simulink model "InverseKinematicsRefMod"  (R2016b)
settings: Solver=VariableStepAuto  StartTime=0.0  StopTime=10.0  RelTol=1e-3
settings Model: DataDictionary=DataDictionary.sldd  Creator=lucadelaat  LastModifiedBy=Taeke

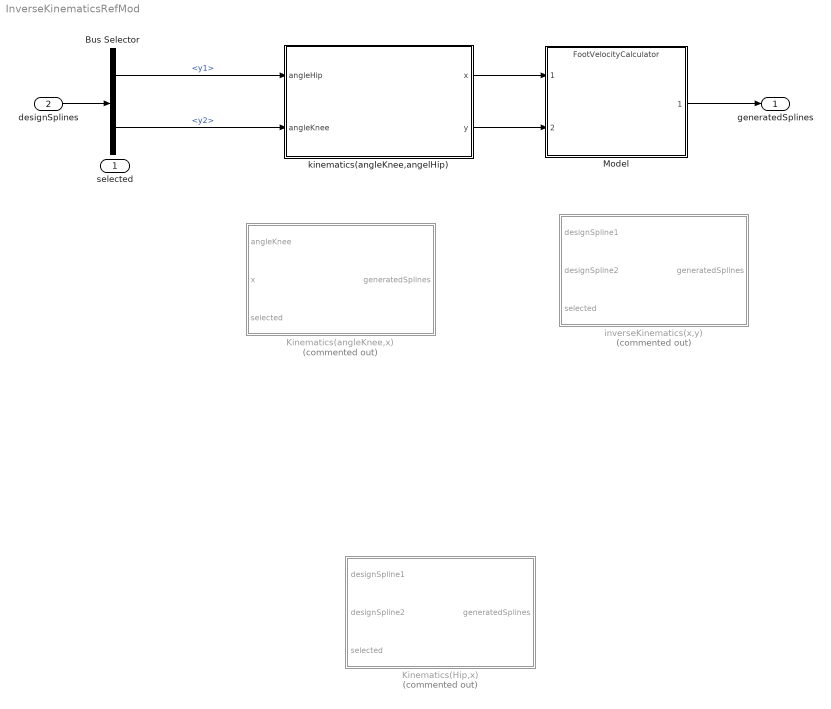
== system InverseKinematicsRefMod ==
  selected : Inport  PortDimensions=4
  designSplines : Inport  Port=2  OutDataTypeStr=Bus: designSplineTotal
  Bus Selector : BusSelector  OutputSignals=designSpline1.y1,designSpline2.y2
  Kinematics(Hip,x) : MATLAB Function  Commented=on  TreatAsAtomicUnit=on
  Kinematics(angleKnee,x) : MATLAB Function  Commented=on  TreatAsAtomicUnit=on
  Model : ModelReference  ModelNameDialog=FootVelocityCalculator.slx  SimulationMode=Normal  ModelReferenceVersion=1.16
  inverseKinematics(x,y) : MATLAB Function  Commented=on  TreatAsAtomicUnit=on
  kinematics(angleKnee,angelHip) : MATLAB Function  TreatAsAtomicUnit=on
  generatedSplines : Outport  OutDataTypeStr=Bus: generatedSplines
  wires:
  designSplines/1 -> Bus Selector/1
  Bus Selector/1 -> kinematics(angleKnee,angelHip)/1(angleHip)  "<y1>"
  Bus Selector/2 -> kinematics(angleKnee,angelHip)/2(angleKnee)  "<y2>"
  kinematics(angleKnee,angelHip)/1(x) -> Model/1
  kinematics(angleKnee,angelHip)/2(y) -> Model/2
  Model/1 -> generatedSplines/1

== matlab function InverseKinematicsRefMod/kinematics(angleKnee,angelHip) ==
  data: angleHip input; angleKnee input; x output; y output
function [x,y] = inverseKinematics(angleHip,angleKnee)
Lul = 0.4; %[m] Length upper leg (no not of something else)
Lll = 0.4; %[m] Length lower leg

x1 = Lul*sin(angleHip);
y1 = Lul*cos(angleHip);

x2 = -Lll*cos(0.5*pi+angleHip - angleKnee);
y2 = Lll*sin(0.5*pi+angleHip - angleKnee);

x = x1+x2;
y = Lul + Lll - y2 - y1;
end

== matlab function InverseKinematicsRefMod/inverseKinematics(x,y) ==
  data: designSpline1 input; designSpline2 input; generatedSplines output; selected input
function generatedSplines = inverseKinematics(designSpline1,designSpline2, selected)
generatedSplines = 0;
end

== matlab function InverseKinematicsRefMod/Kinematics(angleKnee,x) ==
  data: angleKnee input; x input; generatedSplines output; selected input
function generatedSplines = inverseKinematics(angleKnee,x, selected)
generatedSplines = 0;
end

== matlab function InverseKinematicsRefMod/Kinematics(Hip,x) ==
  data: designSpline1 input; designSpline2 input; generatedSplines output; selected input
function generatedSplines = inverseKinematics(designSpline1,designSpline2, selected)
generatedSplines = 0;
end
